simulink model "Geartrain_Testrig"  (Simulink 7.9)
settings: Solver=ode15s  StartTime=0.0  StopTime=100  RelTol=1e-3
PostLoadFcn:
  | warning off Simulink:Engine:OutputNotConnected
  | warning off Simulink:Engine:UsingDefaultMaxStepSize
  | set_param(gcs,'AlgebraicLoopMsg','none');
undefined symbols (not defined in the file): radps2rpm
libraries: fl_lib x5, nesl_utility x3, Geartrain_Lib x1
Description:
  | Copyright 2011 MathWorks, Inc.
settings Model: Creator=smiller  LastModifiedBy=smiller
settings DebuggingCC: AlgebraicLoopMsg=none  FcnCallInpInsideContextMsg=Use local settings  StrictBusMsg=Warning
settings GRTTargetCC: CombineOutputUpdateFcns=off  GRTInterface=on

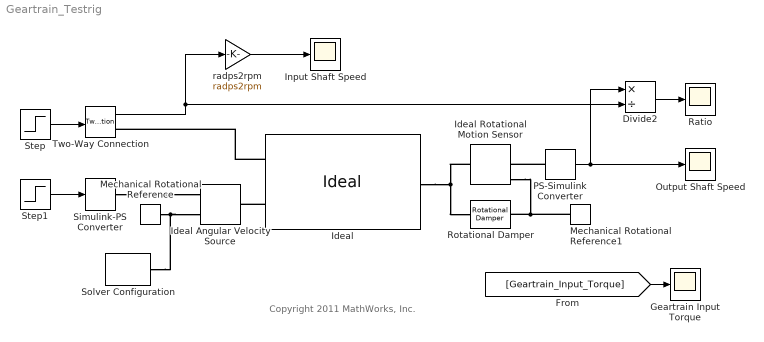
== system Geartrain_Testrig ==
  note: Copyright 2011 MathWorks, Inc.
  Divide2 : Product  Inputs=*/
  Geartrain Input Torque : Scope
      settings: TimeRange=100  YMin=83  YMax=85.5
  Ideal : Geartrain_Lib/Ideal  SystemSampleTime=-1
  Ideal Angular Velocity Source : fl_lib/Mechanical/Mechanical Sources/Ideal Angular Velocity Source  w_Log=off  t_Log=off  LocalVarNames=|w|t  LocalVarDescs=|w|t  LocalVarLogging=[0 0]
  Ideal Rotational Motion Sensor : fl_lib/Mechanical/Mechanical Sensors/Ideal Rotational Motion Sensor  offset=0 rad  w_Log=off  t_Log=off  phi_Log=off  LocalVarNames=|w|t|phi  LocalVarDescs=|w|t|phi  LocalVarLogging=[0 0 0]
  Input Shaft Speed : Scope
      settings: TimeRange=100  YMin=8.5  YMax=11  SaveName=ScopeData6
  Mechanical Rotational Reference : fl_lib/Mechanical/Rotational Elements/Mechanical Rotational Reference  t_Log=off  LocalVarNames=|t  LocalVarDescs=|t  LocalVarLogging=0
  Mechanical Rotational Reference1 : fl_lib/Mechanical/Rotational Elements/Mechanical Rotational Reference  t_Log=off  LocalVarNames=|t  LocalVarDescs=|t  LocalVarLogging=0
  Output Shaft Speed : Scope
      settings: TimeRange=100  YMin=83  YMax=85.5
  PS-Simulink Converter : nesl_utility/PS-Simulink Converter  PhysicalDomain=network_engine_domain  LeftPortType=input  RightPortType=output  SubClassName=ps_output  Unit=1  AffineConversion=off
  Ratio : Scope
      settings: TimeRange=100  YMin=83  YMax=85.5  SaveName=ScopeData5
  Rotational Damper : fl_lib/Mechanical/Rotational Elements/Rotational Damper  D=100 N*m/(rad/s)  t_Log=off  w_Log=off  LocalVarNames=|t|w  LocalVarDescs=|t|w  LocalVarLogging=[0 0]
  Simulink-PS Converter : nesl_utility/Simulink-PS Converter  PhysicalDomain=network_engine_domain  LeftPortType=input  RightPortType=output  SubClassName=ps_input  Unit=1  AffineConversion=off  InputFilterTimeConstant=.001  UdotUserProvided=0  SimscapeFilterOrder=1  InputFiltering=off
  Solver Configuration : nesl_utility/Solver Configuration  PhysicalDomain=network_engine_domain  LeftPortType=input  RightPortType=generic  SubClassName=solver  UseCustomDae=off  DoDC=off  ResidualTolerance=1e-9  UseLocalSolver=off  LocalSolverChoice=NE_BACKWARD_EULER_ADVANCER  LocalSolverSampleTime=.001  DoFixedCost=off  MaxNonlinIter=3  MaxModeIter=2  LinearAlgebra=Sparse  Accelerate=off  Profile=off  UseLocalSampling=off  DelaysMemoryBudget=1024
  Step : Step  Time=5  Before=1  After=0  SampleTime=0
  Step1 : Step  SampleTime=0
  Two-Way Connection : TwoWayConnection
  radps2rpm : Gain  Gain=radps2rpm
  wires:
  Divide2/1 -> Ratio/1
  PS-Simulink Converter/1 -> Divide2/1, Output Shaft Speed/1
  Two-Way Connection/1 -> radps2rpm/1, Divide2/2
  radps2rpm/1 -> Input Shaft Speed/1
  Step/1 -> Two-Way Connection/1
  Step1/1 -> Simulink-PS Converter/1
  [Geartrain_Input_Torque] -> Geartrain Input Torque/1
  connections:
  Ideal/LConn1 -- Two-Way Connection/RConn1
  Simulink-PS Converter/RConn1 -- Ideal Angular Velocity Source/RConn1
  Mechanical Rotational Reference/LConn1 -- Ideal Angular Velocity Source/RConn2 -- Solver Configuration/RConn1
  Mechanical Rotational Reference1/LConn1 -- Rotational Damper/RConn1 -- Ideal Rotational Motion Sensor/RConn1
  Ideal/RConn1 -- Ideal Rotational Motion Sensor/LConn1 -- Rotational Damper/LConn1
  PS-Simulink Converter/LConn1 -- Ideal Rotational Motion Sensor/RConn2
  Ideal/LConn2 -- Ideal Angular Velocity Source/LConn1
